simulink model "Robot"  (Simulink 7.1)
settings: Solver=ode45  StartTime=0.0  StopTime=10.0  RelTol=1e-3
values from neighbouring files (symbols this model uses):
  ADAMS_cwd = '/home/roland/Bureau/Simulateur/SimulateurAdamsFaizRobuFASTB2'    [Controls_Plant_1.m]
  ADAMS_exec = ''    [Controls_Plant_1.m]
  ADAMS_host = 'krid.isir.upmc.fr'    [Controls_Plant_1.m]
  ADAMS_init = ''    [Controls_Plant_1.m]
  ADAMS_inputs = 'AngleBraquageAV!AngleBraquageArriere!AccelMoteur!Stab_function'    [Controls_Plant_1.m]
  ADAMS_outputs = 'PosX!PosY!PosXAvant!PosYAvant!MesureVitesse!AngleAVG!AngleAVD!AngleARG!AngleARD!VitesseRoueARD!VitesseRoueARG!VitesseLacet!roulis'    [Controls_Plant_1.m]
  ADAMS_prefix = 'Controls_Plant_1'    [Controls_Plant_1.m]
  ADAMS_static = 'yes'    [Controls_Plant_1.m]
  ADAMS_sysdir = '/home/roland/Adams/'    [Controls_Plant_1.m]
  C = ParDyn(9)    [MvtDyn.m]    (also in ParPneu.m = 1.3; Replay.m = line([X_trac(6) X_trac(8)],[Y_trac(6) Y_trac(8)],'LineWidth')
settings Model: Creator=roland  LastModifiedBy=roland
settings HardwareCC: ProdHWDeviceType=Generic->Unspecified (assume 32-bit Generic)

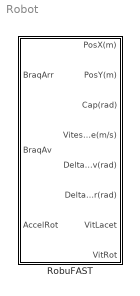
== system Robot ==
  RobuFAST : Subsystem

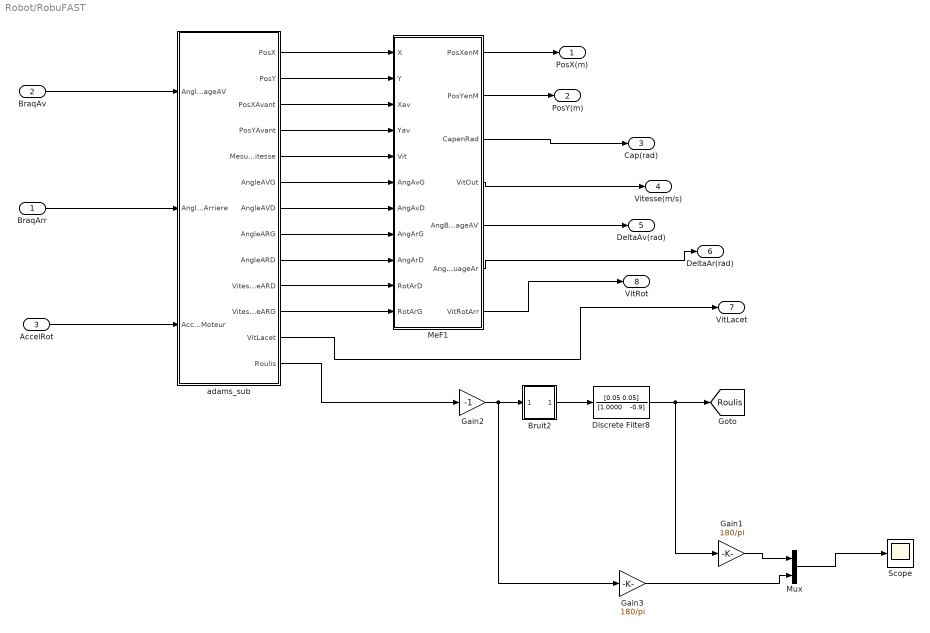
== system Robot/RobuFAST ==
  BraqArr : Inport  OutDataType=sfix(16)  OutScaling=2^0
  BraqAv : Inport  Port=2  OutDataType=sfix(16)  OutScaling=2^0
  AccelRot : Inport  Port=3  OutDataType=sfix(16)  OutScaling=2^0
  Bruit2 : Subsystem
  Discrete Filter8 : DiscreteFilter  Numerator=[0.05 0.05]  Denominator="[1.0000    -0.9]"  SampleTime=0.05
  Gain1 : Gain  Gain=180/pi  ParameterDataType=sfix(16)  ParameterScaling=2^0  OutDataType=sfix(16)  OutScaling=2^0
  Gain2 : Gain  Gain=-1  ParameterDataType=sfix(16)  ParameterScaling=2^0  OutDataType=sfix(16)  OutScaling=2^0
  Gain3 : Gain  Gain=180/pi  ParameterDataType=sfix(16)  ParameterScaling=2^0  OutDataType=sfix(16)  OutScaling=2^0
  MeF1 : Subsystem
  Mux : Mux  Inputs=2
  Scope : Scope
      settings: TimeRange=10  YMin=-0.25  YMax=4.5
  adams_sub : Subsystem
  PosX(m) : Outport  OutDataType=sfix(16)  OutScaling=2^0
  PosY(m) : Outport  Port=2  OutDataType=sfix(16)  OutScaling=2^0
  Cap(rad) : Outport  Port=3  OutDataType=sfix(16)  OutScaling=2^0
  Vitesse(m/s) : Outport  Port=4  OutDataType=sfix(16)  OutScaling=2^0
  DeltaAv(rad) : Outport  Port=5  OutDataType=sfix(16)  OutScaling=2^0
  DeltaAr(rad) : Outport  Port=6  OutDataType=sfix(16)  OutScaling=2^0
  VitLacet : Outport  Port=7  OutDataType=sfix(16)  OutScaling=2^0
  VitRot : Outport  Port=8  OutDataType=sfix(16)  OutScaling=2^0
  tag scope: Roulis=global
  wires:
  MeF1/1(PosXenM) -> PosX(m)/1
  BraqAv/1 -> adams_sub/1("AngleBraquageAV     ")
  MeF1/2(PosYenM) -> PosY(m)/1
  MeF1/4(VitOut) -> Vitesse(m/s)/1
  BraqArr/1 -> adams_sub/2(AngleBraquageArriere)
  MeF1/5(AngBraquageAV) -> DeltaAv(rad)/1
  MeF1/6(AngBraquageAr) -> DeltaAr(rad)/1
  AccelRot/1 -> adams_sub/3("AccelMoteur         ")
  MeF1/7(VitRotArr) -> VitRot/1
  adams_sub/12("VitLacet         ") -> VitLacet/1
  adams_sub/1("PosX             ") -> MeF1/1(X)
  adams_sub/2("PosY             ") -> MeF1/2(Y)
  adams_sub/3("PosXAvant        ") -> MeF1/3(Xav)
  adams_sub/4("PosYAvant        ") -> MeF1/4(Yav)
  adams_sub/5("MesureVitesse    ") -> MeF1/5(Vit)
  adams_sub/6("AngleAVG         ") -> MeF1/6(AngAvG)
  adams_sub/7("AngleAVD         ") -> MeF1/7(AngAvD)
  adams_sub/8("AngleARG         ") -> MeF1/8(AngArG)
  adams_sub/9("AngleARD         ") -> MeF1/9(AngArD)
  adams_sub/10(VitesseAngRoueARD) -> MeF1/10(RotArD)
  adams_sub/11(VitesseAngRoueARG) -> MeF1/11(RotArG)
  MeF1/3(CapenRad) -> Cap(rad)/1
  adams_sub/13("Roulis           ") -> Gain2/1
  Gain2/1 -> Bruit2/1(In1), Gain3/1
  Bruit2/1(Out1) -> Discrete Filter8/1
  Discrete Filter8/1 -> [Roulis], Gain1/1
  Gain1/1 -> Mux/1
  Mux/1 -> Scope/1
  Gain3/1 -> Mux/2

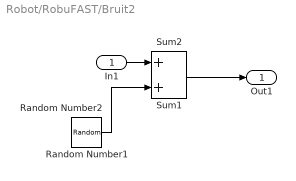
== system Robot/RobuFAST/Bruit2 ==
  In1 : Inport  OutDataType=sfix(16)  OutScaling=2^0
  Random Number1 : RandomNumber  Mean=4*pi/180  Variance=((5/3)*pi/180)^2  Seed=15  SampleTime=0.05
  Random Number2 : RandomNumber  Variance=0.0007  SampleTime=0.025
  Sum1 : Sum  OutDataType=sfix(16)  OutScaling=2^0
  Sum2 : Sum  OutDataType=sfix(16)  OutScaling=2^0
  Out1 : Outport  OutDataType=sfix(16)  OutScaling=2^0
  wires:
  Sum1/1 -> Out1/1
  In1/1 -> Sum1/1
  Random Number2/1 -> Sum1/2

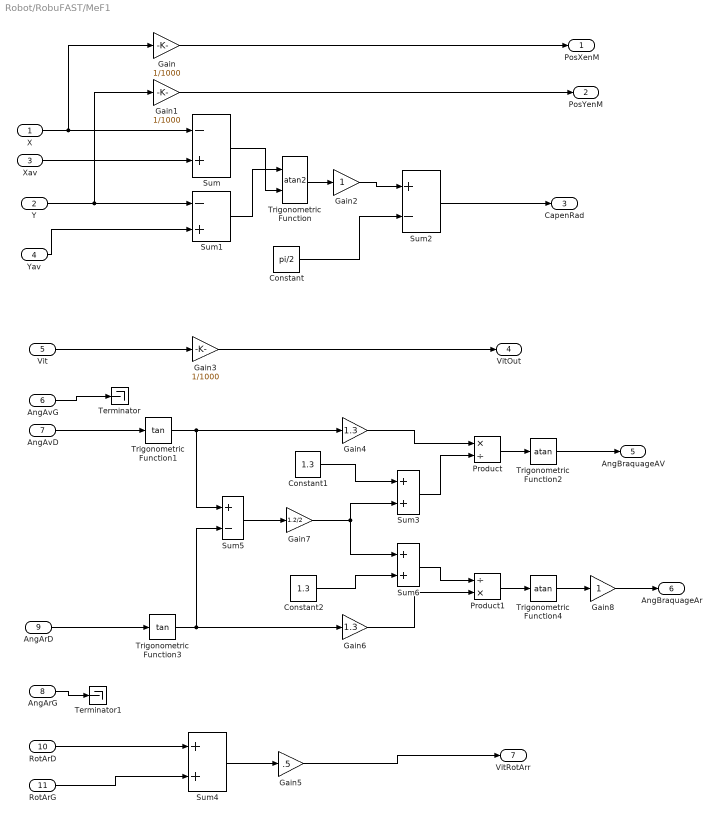
== system Robot/RobuFAST/MeF1 ==
  X : Inport  OutDataType=sfix(16)  OutScaling=2^0
  Y : Inport  Port=2  OutDataType=sfix(16)  OutScaling=2^0
  Xav : Inport  Port=3  OutDataType=sfix(16)  OutScaling=2^0
  Yav : Inport  Port=4  OutDataType=sfix(16)  OutScaling=2^0
  Vit : Inport  Port=5  OutDataType=sfix(16)  OutScaling=2^0
  AngAvG : Inport  Port=6  OutDataType=sfix(16)  OutScaling=2^0
  AngAvD : Inport  Port=7  OutDataType=sfix(16)  OutScaling=2^0
  AngArG : Inport  Port=8  OutDataType=sfix(16)  OutScaling=2^0
  AngArD : Inport  Port=9  OutDataType=sfix(16)  OutScaling=2^0
  RotArD : Inport  Port=10  OutDataType=sfix(16)  OutScaling=2^0
  RotArG : Inport  Port=11  OutDataType=sfix(16)  OutScaling=2^0
  Constant : Constant  Value=pi/2  OutDataType=sfix(16)  OutScaling=2^0
  Constant1 : Constant  Value=1.3  OutDataType=sfix(16)  OutScaling=2^0
  Constant2 : Constant  Value=1.3  OutDataType=sfix(16)  OutScaling=2^0
  Gain : Gain  Gain=1/1000  ParameterDataType=sfix(16)  ParameterScaling=2^0  OutDataType=sfix(16)  OutScaling=2^0
  Gain1 : Gain  Gain=1/1000  ParameterDataType=sfix(16)  ParameterScaling=2^0  OutDataType=sfix(16)  OutScaling=2^0
  Gain2 : Gain  ParameterDataType=sfix(16)  ParameterScaling=2^0  OutDataType=sfix(16)  OutScaling=2^0
  Gain3 : Gain  Gain=1/1000  ParameterDataType=sfix(16)  ParameterScaling=2^0  OutDataType=sfix(16)  OutScaling=2^0
  Gain4 : Gain  Gain=1.3  ParameterDataType=sfix(16)  ParameterScaling=2^0  OutDataType=sfix(16)  OutScaling=2^0
  Gain5 : Gain  Gain=.5  ParameterDataType=sfix(16)  ParameterScaling=2^0  OutDataType=sfix(16)  OutScaling=2^0
  Gain6 : Gain  Gain=1.3  ParameterDataType=sfix(16)  ParameterScaling=2^0  OutDataType=sfix(16)  OutScaling=2^0
  Gain7 : Gain  Gain=1.2/2  ParameterDataType=sfix(16)  ParameterScaling=2^0  OutDataType=sfix(16)  OutScaling=2^0
  Gain8 : Gain  ParameterDataType=sfix(16)  ParameterScaling=2^0  OutDataType=sfix(16)  OutScaling=2^0
  Product : Product  Inputs=*/  OutDataType=sfix(16)  OutScaling=2^0  RndMeth=Zero
  Product1 : Product  Inputs=/*  OutDataType=sfix(16)  OutScaling=2^0  RndMeth=Zero
  Sum : Sum  Inputs=-+  OutDataType=sfix(16)  OutScaling=2^0
  Sum1 : Sum  Inputs=-+  OutDataType=sfix(16)  OutScaling=2^0
  Sum2 : Sum  Inputs=+-  OutDataType=sfix(16)  OutScaling=2^0
  Sum3 : Sum  OutDataType=sfix(16)  OutScaling=2^0
  Sum4 : Sum  OutDataType=sfix(16)  OutScaling=2^0
  Sum5 : Sum  Inputs=+-  OutDataType=sfix(16)  OutScaling=2^0
  Sum6 : Sum  OutDataType=sfix(16)  OutScaling=2^0
  Terminator : Terminator
  Terminator1 : Terminator
  Trigonometric Function : Trigonometry  Operator=atan2
  Trigonometric Function1 : Trigonometry  Operator=tan
  Trigonometric Function2 : Trigonometry  Operator=atan
  Trigonometric Function3 : Trigonometry  Operator=tan
  Trigonometric Function4 : Trigonometry  Operator=atan
  PosXenM : Outport  OutDataType=sfix(16)  OutScaling=2^0
  PosYenM : Outport  Port=2  OutDataType=sfix(16)  OutScaling=2^0
  CapenRad : Outport  Port=3  OutDataType=sfix(16)  OutScaling=2^0
  VitOut : Outport  Port=4  OutDataType=sfix(16)  OutScaling=2^0
  AngBraquageAV : Outport  Port=5  OutDataType=sfix(16)  OutScaling=2^0
  AngBraquageAr : Outport  Port=6  OutDataType=sfix(16)  OutScaling=2^0
  VitRotArr : Outport  Port=7  OutDataType=sfix(16)  OutScaling=2^0
  wires:
  X/1 -> Sum/1, Gain/1
  Y/1 -> Sum1/1, Gain1/1
  Xav/1 -> Sum/2
  Trigonometric Function/1 -> Gain2/1
  Yav/1 -> Sum1/2
  Gain1/1 -> PosYenM/1
  Gain2/1 -> Sum2/1
  Constant/1 -> Sum2/2
  Sum2/1 -> CapenRad/1
  Vit/1 -> Gain3/1
  Gain3/1 -> VitOut/1
  AngAvD/1 -> Trigonometric Function1/1
  Sum4/1 -> Gain5/1
  RotArD/1 -> Sum4/1
  RotArG/1 -> Sum4/2
  Gain5/1 -> VitRotArr/1
  AngArD/1 -> Trigonometric Function3/1
  AngAvG/1 -> Terminator/1
  Trigonometric Function1/1 -> Gain4/1, Sum5/1
  Sum3/1 -> Product/2
  Gain4/1 -> Product/1
  Product/1 -> Trigonometric Function2/1
  Trigonometric Function2/1 -> AngBraquageAV/1
  AngArG/1 -> Terminator1/1
  Trigonometric Function3/1 -> Gain6/1, Sum5/2
  Constant1/1 -> Sum3/1
  Sum5/1 -> Gain7/1
  Gain7/1 -> Sum3/2, Sum6/1
  Sum6/1 -> Product1/1
  Gain6/1 -> Product1/2
  Constant2/1 -> Sum6/2
  Product1/1 -> Trigonometric Function4/1
  Trigonometric Function4/1 -> Gain8/1
  Gain8/1 -> AngBraquageAr/1
  Sum1/1 -> Trigonometric Function/1
  Sum/1 -> Trigonometric Function/2
  Gain/1 -> PosXenM/1

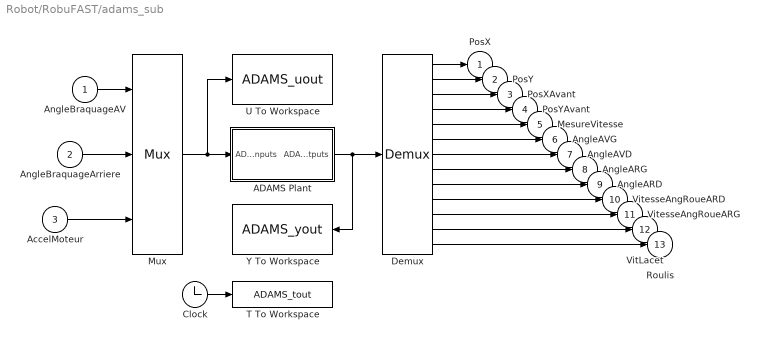
== system Robot/RobuFAST/adams_sub ==
  "AngleBraquageAV     " : Inport
  AngleBraquageArriere : Inport  Port=2
  "AccelMoteur         " : Inport  Port=3
  ADAMS Plant : Subsystem  mask(Adams Plant){exevie=ADAMS_sysdir, workdir=ADAMS_cwd, comtyp=PIPE(DDE), ada_host=ADAMS_host, exetyp=C++, exesol=ADAMS_exec, nampre=ADAMS_prefix, nam_in=ADAMS_inputs, namout=ADAMS_outputs, outfil=ADAMS_prefix, dt_out=0.005, o_rate=1, interorder=0, dft=no, modsim=discrete, modani=interactive, stat=ADAMS_static, inicmd=[ADAMS_init]}
      mask prompts: exevie "Adams install directory"; workdir "Adams working directory"; comtyp "Interprocess Option"; ada_host "Adams host"; exetyp "Adams solver type"; exesol "User executable (opt.: if blank - use standard)"; nampre "Adams model file prefix"; nam_in "Adams/View input names"; namout "Adams/View output names"; outfil "Output files prefix (opt.: if blank - no output)"; dt_out "Communication Interval"; o_rate "Number of communications per output step"; interorder "Interpolation Order"; dft "Direct Feedthrough"; modsim "Simulation     mode"; modani "Animation     mode"; stat "Initial Static Simulation Flag"; inicmd "Initialization commands"
      mask help: Simulate any Adams plant model either in Adams/Solver form (.adm file) or in Adams/View form (.cmd file)
      mask StyleString: edit,edit,popup(PIPE(DDE)|TCP/IP),edit,popup(Fortran|C++),edit,edit,edit,edit,edit,edit,edit,edit,popup(no|yes),popup(discrete|continuous),popup(batch|interactive),edit,edit
      mask Display: disp( 'MSCSoftware' )
  Clock : Clock
      settings: Decimation=10
  Demux : Demux  Outputs=13
  Mux : Mux  Inputs=3
  T To Workspace : ToWorkspace  VariableName=ADAMS_tout  SaveFormat=Array
      settings: MaxDataPoints=100000
  U To Workspace : ToWorkspace  VariableName=ADAMS_uout  SaveFormat=Array
      settings: MaxDataPoints=100000
  Y To Workspace : ToWorkspace  VariableName=ADAMS_yout  SaveFormat=Array
      settings: MaxDataPoints=100000
  "PosX             " : Outport
  "PosY             " : Outport  Port=2
  "PosXAvant        " : Outport  Port=3
  "PosYAvant        " : Outport  Port=4
  "MesureVitesse    " : Outport  Port=5
  "AngleAVG         " : Outport  Port=6
  "AngleAVD         " : Outport  Port=7
  "AngleARG         " : Outport  Port=8
  "AngleARD         " : Outport  Port=9
  VitesseAngRoueARD : Outport  Port=10
  VitesseAngRoueARG : Outport  Port=11
  "VitLacet         " : Outport  Port=12
  "Roulis           " : Outport  Port=13
  wires:
  Clock/1 -> T To Workspace/1
  Mux/1 -> ADAMS Plant/1(ADAMS inputs), U To Workspace/1
  ADAMS Plant/1(ADAMS outputs) -> Demux/1, Y To Workspace/1
  Demux/1 -> "PosX             "/1
  Demux/2 -> "PosY             "/1
  Demux/3 -> "PosXAvant        "/1
  Demux/4 -> "PosYAvant        "/1
  Demux/5 -> "MesureVitesse    "/1
  Demux/6 -> "AngleAVG         "/1
  Demux/7 -> "AngleAVD         "/1
  Demux/8 -> "AngleARG         "/1
  Demux/9 -> "AngleARD         "/1
  Demux/10 -> VitesseAngRoueARD/1
  Demux/11 -> VitesseAngRoueARG/1
  Demux/12 -> "VitLacet         "/1
  Demux/13 -> "Roulis           "/1
  "AngleBraquageAV     "/1 -> Mux/1
  AngleBraquageArriere/1 -> Mux/2
  "AccelMoteur         "/1 -> Mux/3

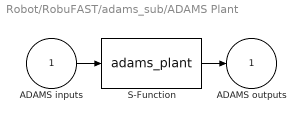
== system Robot/RobuFAST/adams_sub/ADAMS Plant ==
  ADAMS inputs : Inport
  S-Function : S-Function  FunctionName=adams_plant  Parameters=exevie,exesol,stat,outfil,nampre,o_rate,nam_in,namout,dft,modsim,modani,dt_out,inicmd,exetyp,comtyp,ada_host, workdir,interorder  EnableBusSupport=off
  ADAMS outputs : Outport  InitialOutput=0
  wires:
  ADAMS inputs/1 -> S-Function/1
  S-Function/1 -> ADAMS outputs/1
